simulink model "batt_electrics_RUL_SOC"  (R2022a)
settings: Solver=FixedStepAuto  StartTime=0.0  StopTime=1800*100  FixedStep=1e-1  RelTol=1e-3
undefined symbols (not defined in the file or in its folder): DiscIntNeverNeededParam
libraries: ee_lib x16, nesl_utility x6, fl_lib x4, simulink x1, dspstat3 x1
(part 3 of 3)

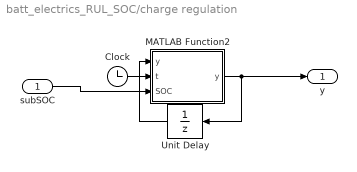
== system batt_electrics_RUL_SOC/charge regulation ==
  subSOC : Inport
  Clock : Clock
  MATLAB Function2 : MATLAB Function  TreatAsAtomicUnit=on
  Unit Delay : UnitDelay  InitialCondition=-1  SampleTime=-1  HasFrameUpgradeWarning=on
  y : Outport
  wires:
  MATLAB Function2/1(y) -> Unit Delay/1, y/1
  Unit Delay/1 -> MATLAB Function2/1("y ")
  Clock/1 -> MATLAB Function2/2(t)
  subSOC/1 -> MATLAB Function2/3(SOC)

== matlab function batt_electrics_RUL_SOC/charge regulation/MATLAB Function2 ==
  data: y input; y output; t input; SOC input
function y = fcn(y,t, SOC)
    interval = 1800;

    if  rem(t, interval) == 0 || SOC == 0.3
        y=300; 
    end
        if SOC>=1
            y=-1;% Assigning 100 to the first element of y if the condition is met
        % Assigning -1 to the first element of y if SOC is 1
    end
end
